simulink model "SyncGen_with_omega_V_controll_two_generators_oceilations"  (R2013a)
settings: Solver=ode45  StartTime=5  StopTime=10  FixedStep=10^-3  MaxStep=10^-3  RelTol=1e-5
undefined symbols (not defined in the file): J
libraries: powerlib x8, powerlib_meascontrol x3, ControledSyncGenLib x2
settings Model: Creator=Elad  LastModifiedBy=USER
settings DataIOCC: SignalLoggingSaveFormat=ModelDataLogs
settings DebuggingCC: MultiTaskDSMMsg=warning  MultiTaskCondExecSysMsg=none  StateNameClashWarn=none  StrictBusMsg=None
settings RTWCC: IncludeERTFirstTime=on

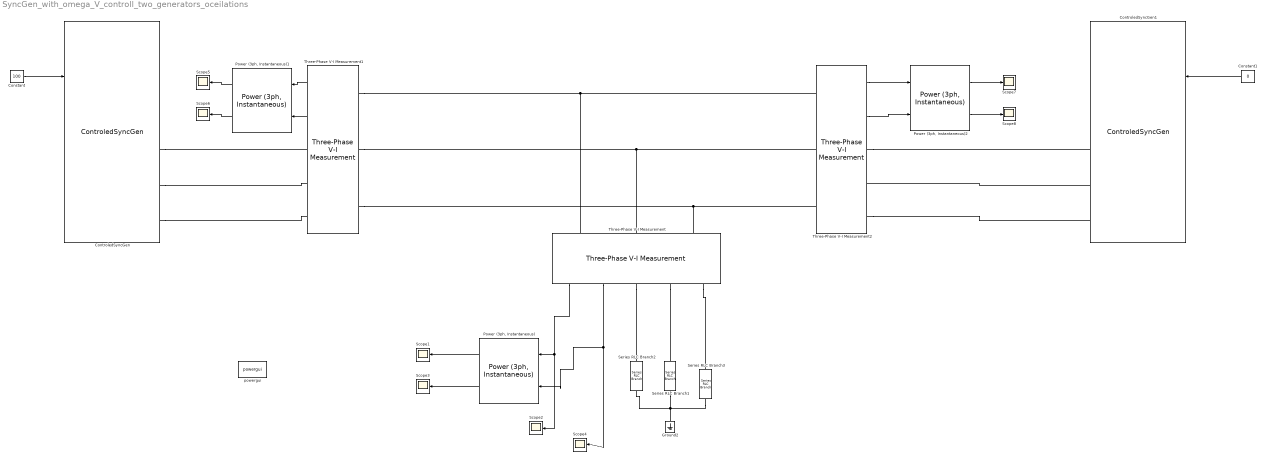
== system SyncGen_with_omega_V_controll_two_generators_oceilations ==
  Constant : Constant  Value=100
  Constant1 : Constant  Value=0
  ControledSyncGen : ControledSyncGenLib/ControledSyncGen  R_f=R_f  R_s=R_s  D_p=D_p  J=J  M_f=M_f  L_f=L_f  L_s=L_s  K_p=0.2  D_q=20  K=1
      link override Gain1: Gain=1/(2*pi*50)
      link override Gain4: Gain=1/K
  ControledSyncGen1 : ControledSyncGenLib/ControledSyncGen  R_f=R_f  R_s=R_s  D_p=D_p  J=J  M_f=M_f  L_f=L_f  L_s=L_s  K_p=0.2  D_q=20  K=1
      link override Gain1: Gain=1/(2*pi*50)
      link override Gain4: Gain=1/K
  Ground2 : powerlib/Elements/Ground  LConnTagsString=a
  "Power (3ph, Instantaneous)" : powerlib_meascontrol/Measurements/Power (3ph, Instantaneous)
  "Power (3ph, Instantaneous)1" : powerlib_meascontrol/Measurements/Power (3ph, Instantaneous)
  "Power (3ph, Instantaneous)2" : powerlib_meascontrol/Measurements/Power (3ph, Instantaneous)
  Scope{1..8} (8 alike) : Scope
      Scope1 settings: TimeRange=5  YMin=54.2787  YMax=54.2798
      Scope2 settings: TimeRange=5  YMin=-275  YMax=275
      Scope3 settings: TimeRange=5  YMin=-225  YMax=225  SaveName=ScopeData3
      Scope4 settings: TimeRange=5  YMin=-0.005  YMax=0.005  SaveName=ScopeData4
      Scope5 settings: TimeRange=5  YMin=-27.1399  YMax=-27.1394  SaveName=ScopeData2
      Scope6 settings: TimeRange=5  YMin=-225  YMax=225  SaveName=ScopeData5
      Scope7 settings: TimeRange=5  YMin=-27.1403  YMax=-27.1394  SaveName=ScopeData6
      Scope8 settings: TimeRange=5  YMin=-225  YMax=225  SaveName=ScopeData7
  Series RLC Branch1 : powerlib/Elements/Series RLC Branch  LConnTagsString=__new0  RConnTagsString=__new0  BranchType=R  Resistance=1000  Inductance=1e-3  SetiL0=off  InitialCurrent=0  Capacitance=1e-6  Setx0=off  InitialVoltage=0  Measurements=None
  Series RLC Branch2 : powerlib/Elements/Series RLC Branch  LConnTagsString=__new0  RConnTagsString=__new0  BranchType=R  Resistance=1000  Inductance=1e-3  SetiL0=off  InitialCurrent=0  Capacitance=1e-6  Setx0=off  InitialVoltage=0  Measurements=None
  Series RLC Branch3 : powerlib/Elements/Series RLC Branch  LConnTagsString=__new0  RConnTagsString=__new0  BranchType=R  Resistance=1000  Inductance=1e-3  SetiL0=off  InitialCurrent=0  Capacitance=1e-6  Setx0=off  InitialVoltage=0  Measurements=None
  Three-Phase V-I Measurement : powerlib/Measurements/Three-Phase V-I Measurement  VoltageMeasurement=phase-to-ground  SetLabelV=off  LabelV=Vabc  Vpu=off  VpuLL=off  CurrentMeasurement=yes  SetLabelI=off  LabelI=Iabc  Ipu=off  Pbase=100e6  Vbase=500e3  OutputType=Complex  PhasorSimulation=off  PSBequivalent=0
  Three-Phase V-I Measurement1 : powerlib/Measurements/Three-Phase V-I Measurement  VoltageMeasurement=phase-to-ground  SetLabelV=off  LabelV=Vabc  Vpu=off  VpuLL=off  CurrentMeasurement=yes  SetLabelI=off  LabelI=Iabc  Ipu=off  Pbase=100e6  Vbase=500e3  OutputType=Complex  PhasorSimulation=off  PSBequivalent=0
  Three-Phase V-I Measurement2 : powerlib/Measurements/Three-Phase V-I Measurement  VoltageMeasurement=phase-to-ground  SetLabelV=off  LabelV=Vabc  Vpu=off  VpuLL=off  CurrentMeasurement=yes  SetLabelI=off  LabelI=Iabc  Ipu=off  Pbase=100e6  Vbase=500e3  OutputType=Complex  PhasorSimulation=off  PSBequivalent=0
  powergui : powerlib/powergui  Priority=1  SimulationMode=Continuous  SolverType=Tustin  SampleTime=50e-6  frequency=60  SPID=off  DisableSnubberDevices=off  DisableRonSwitches=off  DisableVfSwitches=off  SwTol=0  Interpol=off  DisplayEquations=off  frequencyindice=0  Pbase=100e6  ErrMax=1e-4  Iterations=50  UnitsV=kV  UnitsW=MW  FunctionMessages=off  echomessages=off  HookPort=off  EnableUseOfTLC=off  x0status=blocks  RestoreLinks=warning  ResistiveCurrentMeasurement=off  Frange=[0:2:500]  Ylog=off  Xlog=on  ShowGrid=off  save=off  variable=ZData  ZoomFFT=off  StartTime=0.0  cycles=1  DisplayStyle=1  fundamental=60  FreqAxis=off  MaxFrequency=1000  frequencyindicesteady=1  RmsSteady=1  display=off  Ts=0  methode=off
  wires:
  "Power (3ph, Instantaneous)"/1 -> Scope1/1
  "Power (3ph, Instantaneous)"/2 -> Scope3/1
  Three-Phase V-I Measurement/1 -> Scope2/1, "Power (3ph, Instantaneous)"/1
  Three-Phase V-I Measurement/2 -> "Power (3ph, Instantaneous)"/2, Scope4/1
  Three-Phase V-I Measurement1/2 -> "Power (3ph, Instantaneous)1"/2
  Three-Phase V-I Measurement1/1 -> "Power (3ph, Instantaneous)1"/1
  "Power (3ph, Instantaneous)1"/1 -> Scope5/1
  "Power (3ph, Instantaneous)1"/2 -> Scope6/1
  Three-Phase V-I Measurement2/1 -> "Power (3ph, Instantaneous)2"/1
  Three-Phase V-I Measurement2/2 -> "Power (3ph, Instantaneous)2"/2
  "Power (3ph, Instantaneous)2"/2 -> Scope8/1
  "Power (3ph, Instantaneous)2"/1 -> Scope7/1
  Constant/1 -> ControledSyncGen/1
  Constant1/1 -> ControledSyncGen1/1
  connections:
  Series RLC Branch3/RConn1 -- Series RLC Branch2/RConn1 -- Ground2/LConn1 -- Series RLC Branch1/RConn1
  Three-Phase V-I Measurement1/LConn1 -- Three-Phase V-I Measurement2/LConn1 -- Three-Phase V-I Measurement/LConn1
  Three-Phase V-I Measurement1/LConn2 -- Three-Phase V-I Measurement2/LConn2 -- Three-Phase V-I Measurement/LConn2
  Three-Phase V-I Measurement1/LConn3 -- Three-Phase V-I Measurement2/LConn3 -- Three-Phase V-I Measurement/LConn3
  Three-Phase V-I Measurement/RConn3 -- Series RLC Branch3/LConn1
  Three-Phase V-I Measurement/RConn2 -- Series RLC Branch1/LConn1
  Three-Phase V-I Measurement/RConn1 -- Series RLC Branch2/LConn1
  ControledSyncGen/RConn1 -- Three-Phase V-I Measurement1/RConn1
  ControledSyncGen/RConn2 -- Three-Phase V-I Measurement1/RConn2
  ControledSyncGen/RConn3 -- Three-Phase V-I Measurement1/RConn3
  Three-Phase V-I Measurement2/RConn3 -- ControledSyncGen1/RConn3
  ControledSyncGen1/RConn2 -- Three-Phase V-I Measurement2/RConn2
  Three-Phase V-I Measurement2/RConn1 -- ControledSyncGen1/RConn1
